simulink model "OPC_Server"  (R2021b)
settings: Solver=VariableStepAuto  StartTime=0.0  StopTime=100.0  RelTol=1e-3
settings Model: Creator=xxjyj  LastModifiedBy=xxjyj

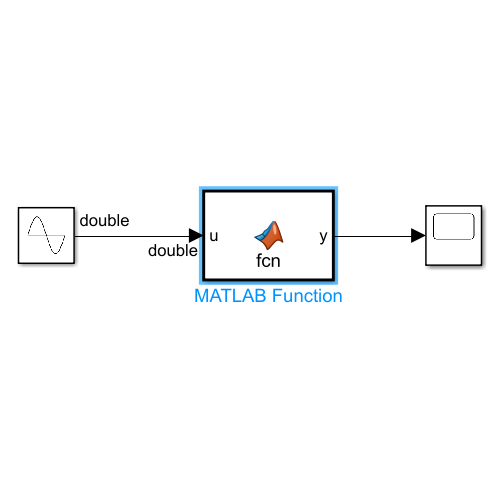
[thumbnail: Simulink's stored preview of the top-level diagram]
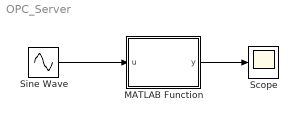
== system OPC_Server ==
  MATLAB Function : MATLAB Function  TreatAsAtomicUnit=on
  Scope : Scope
  Sine Wave : Sin  SampleTime=0
  wires:
  Sine Wave/1 -> MATLAB Function/1(u)
  MATLAB Function/1(y) -> Scope/1

== matlab function OPC_Server/MATLAB Function ==
  data: u input; y output
function y = fcn(u)

coder.extrinsic('opcua');
coder.extrinsic('connect');
coder.extrinsic('opcuanode');
coder.extrinsic('readValue');


persistent ConnectFlag;
if isempty(ConnectFlag)
    ConnectFlag = 0;
end

persistent UaClient;
if isempty(UaClient)
    UaClient = opcua('localhost', 4840);
end

if ConnectFlag == 0
    connect(UaClient);
    ConnectFlag = 1;
end

ClientNode = opcuanode(1, 1, UaClient);
[val, ts, qual] = readValue(UaClient, ClientNode);

y = u;
